simulink model "SIM_CSTR"  (R2023b)
settings: Solver=VariableStepAuto  StartTime=0.0  StopTime=30  RelTol=1e-3
values from neighbouring files (symbols this model uses):
  Ts = 0.05    [NMPC_CSTR.m]
  u0 = 300    [NMPC_CSTR.m]
libraries: sharedTrackingLibrary x1, mpclib x1, simulink x1
settings Model: Creator=DELL  LastModifiedBy=akeebismail

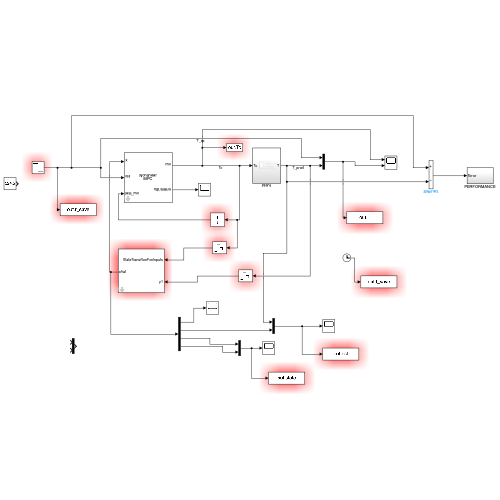
[thumbnail: Simulink's stored preview of the top-level diagram]
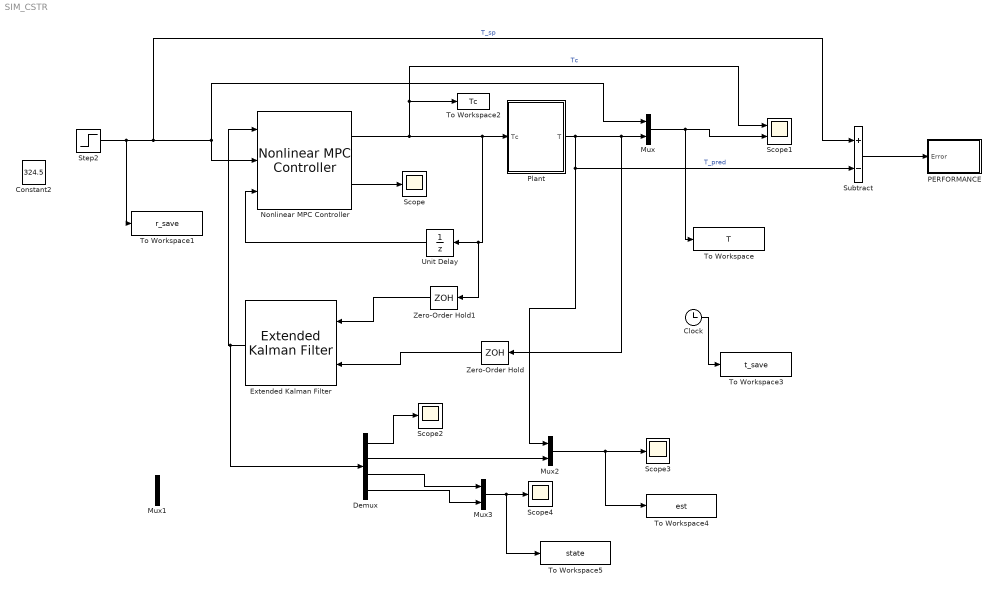
== system SIM_CSTR ==
  Clock : Clock
  Constant2 : Constant  Value=324.5
  Demux : Demux
  Extended Kalman Filter : sharedTrackingLibrary/Extended Kalman Filter  StateTransitionFcn=cstrStateFcnDT  HasStateTransitionJacobianFcn=off  HasAdditiveProcessNoise=Additive  ProcessNoise=[1e-1;1e-1;1e-1;1e-1]  HasTimeVaryingProcessNoise=off  HasStateTransitionFcnExtraArgument=1  InitialState=y0  InitialStateCovariance=[1;1;1;1]  MeasurementFcn1=cstrMeasFcn  HasMeasurementJacobianFcn1=off  HasMeasurementEnablePort1=off  HasAdditiveMeasurementNoise1=Additive  MeasurementNoise1=1e-2  HasTimeVaryingMeasurementNoise1=off  HasMeasurementFcnExtraArgument1=0  HasMeasurementWrapping1=off  MeasurementFcn2=myMeasurementFcn  HasMeasurementJacobianFcn2=off  HasMeasurementEnablePort2=off  HasAdditiveMeasurementNoise2=Additive  MeasurementNoise2=1  HasTimeVaryingMeasurementNoise2=off  HasMeasurementFcnExtraArgument2=0  HasMeasurementWrapping2=off  MeasurementFcn3=myMeasurementFcn  HasMeasurementJacobianFcn3=off  HasMeasurementEnablePort3=off  HasAdditiveMeasurementNoise3=Additive  MeasurementNoise3=1  HasTimeVaryingMeasurementNoise3=off  HasMeasurementFcnExtraArgument3=0  HasMeasurementWrapping3=off  MeasurementFcn4=myMeasurementFcn  HasMeasurementJacobianFcn4=off  HasMeasurementEnablePort4=off  HasAdditiveMeasurementNoise4=Additive  MeasurementNoise4=1  HasTimeVaryingMeasurementNoise4=off  HasMeasurementFcnExtraArgument4=0  HasMeasurementWrapping4=off  MeasurementFcn5=myMeasurementFcn  HasMeasurementJacobianFcn5=off  HasMeasurementEnablePort5=off  HasAdditiveMeasurementNoise5=Additive  MeasurementNoise5=1  HasTimeVaryingMeasurementNoise5=off  HasMeasurementFcnExtraArgument5=0  HasMeasurementWrapping5=off  EnableMultirate=off  StateTransitionFcnSampleTime=1  MeasurementFcn1SampleTime=1  MeasurementFcn2SampleTime=1  MeasurementFcn3SampleTime=1  MeasurementFcn4SampleTime=1  MeasurementFcn5SampleTime=1  UseCurrentEstimator=on  OutputStateCovariance=off  DataType=double  SampleTime=Ts  NumberOfMeasurements=1
  Mux{,1..3} (4 alike) : Mux  Inputs=2
  Nonlinear MPC Controller : mpclib/Nonlinear MPC Controller  nlmpcobj=nlobj  UseObjectTs=on  UseMEX=off  md_enabled=off  mvtarget_enabled=off  param_enabled=off  cost_enabled=off  mvseq_enabled=off  stateseq_enabled=off  ovseq_enabled=off  slack_enabled=off  status_enabled=on  ov_min=off  ov_max=off  mv_min=off  mv_max=off  mvrate_min=off  mvrate_max=off  state_min=off  state_max=off  ov_weight=off  mv_weight=off  mvrate_weight=off  ecr_weight=off  nlp_initialize=off
  PERFORMANCE : Subsystem
  Plant : Subsystem
  Scope{,2..4} (4 alike) : Scope
  Scope1 : Scope  NumInputPorts=2
  Step2 : Step  Time=10  Before=324.5  After=305  SampleTime=Ts
  Subtract : Sum  Inputs=+-
  To Workspace : ToWorkspace  VariableName=T  SaveFormat=Timeseries  SampleTime=Ts
  To Workspace1 : ToWorkspace  VariableName=r_save  SaveFormat=Timeseries  SampleTime=Ts
  To Workspace2 : ToWorkspace  VariableName=Tc  SaveFormat=Timeseries  SampleTime=Ts
  To Workspace3 : ToWorkspace  VariableName=t_save  SaveFormat=Timeseries  SampleTime=Ts
  To Workspace4 : ToWorkspace  VariableName=est  SaveFormat=Timeseries  SampleTime=Ts
  To Workspace5 : ToWorkspace  VariableName=state  SaveFormat=Timeseries  SampleTime=Ts
  Unit Delay : UnitDelay  InitialCondition=u0  SampleTime=Ts  HasFrameUpgradeWarning=on
  Zero-Order Hold : ZeroOrderHold  SampleTime=Ts
  Zero-Order Hold1 : ZeroOrderHold  SampleTime=Ts
  wires:
  Step2/1 -> To Workspace1/1, Subtract/1, Nonlinear MPC Controller/2, Mux/1  "T_sp"
  Nonlinear MPC Controller/1 -> To Workspace2/1, Scope1/1, Plant/1(Tc), Zero-Order Hold1/1, Unit Delay/1  "Tc"
  Plant/1(T) -> Subtract/2, Mux2/1, Zero-Order Hold/1, Mux/2  "T_pred"
  Nonlinear MPC Controller/2 -> Scope/1
  Mux/1 -> To Workspace/1, Scope1/2
  Zero-Order Hold/1 -> Extended Kalman Filter/2
  Unit Delay/1 -> Nonlinear MPC Controller/3
  Zero-Order Hold1/1 -> Extended Kalman Filter/1
  Clock/1 -> To Workspace3/1
  Extended Kalman Filter/1 -> Demux/1, Nonlinear MPC Controller/1
  Demux/2 -> Mux2/2
  Demux/1 -> Scope2/1
  Mux2/1 -> Scope3/1, To Workspace4/1
  Demux/3 -> Mux3/1
  Demux/4 -> Mux3/2
  Mux3/1 -> To Workspace5/1, Scope4/1
  Subtract/1 -> PERFORMANCE/1(Error)

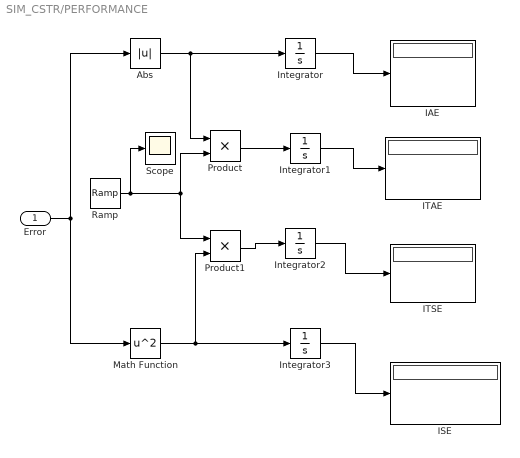
== system SIM_CSTR/PERFORMANCE ==
  Error : Inport
  Abs : Abs  SaturateOnIntegerOverflow=off
  IAE : Display
  ISE : Display
  ITAE : Display
  ITSE : Display
  Integrator{,1..3} (4 alike) : Integrator
  Math Function : Math  Operator=square  SignedPower=on
  Product : Product  RndMeth=Zero
  Product1 : Product  RndMeth=Zero
  Ramp : simulink/Sources/Ramp  slope=1  start=0  InitialOutput=0
  Scope : Scope
  wires:
  Error/1 -> Math Function/1, Abs/1
  Abs/1 -> Integrator/1, Product/1
  Integrator/1 -> IAE/1
  Ramp/1 -> Product/2, Product1/1, Scope/1
  Math Function/1 -> Integrator3/1, Product1/2
  Product1/1 -> Integrator2/1
  Product/1 -> Integrator1/1
  Integrator3/1 -> ISE/1
  Integrator2/1 -> ITSE/1
  Integrator1/1 -> ITAE/1

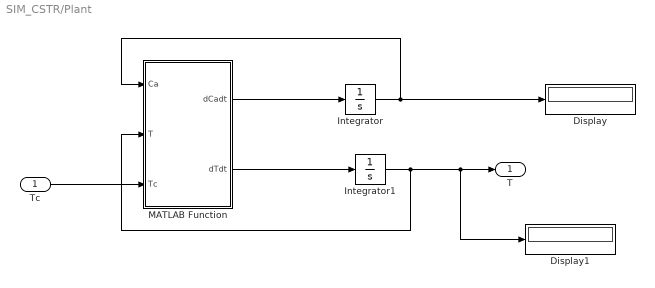
== system SIM_CSTR/Plant ==
  Tc : Inport
  Display : Display
  Display1 : Display
  Integrator : Integrator
  Integrator1 : Integrator  InitialCondition=300
  MATLAB Function : MATLAB Function  TreatAsAtomicUnit=on
  T : Outport
  wires:
  Integrator1/1 -> Display1/1, T/1, MATLAB Function/2(T)
  MATLAB Function/2(dTdt) -> Integrator1/1
  Integrator/1 -> Display/1, MATLAB Function/1(Ca)
  MATLAB Function/1(dCadt) -> Integrator/1
  Tc/1 -> MATLAB Function/3(Tc)

== matlab function SIM_CSTR/Plant/MATLAB Function ==
  data: Ca input; dCadt output; T input; Tc input; dTdt output
function [dCadt,dTdt] = fcn(Ca,T,Tc)

values = {100,5e4,350,100,1000,0.239,8750,7.2e10,5e4,1};
[F,delta_H,Tf,V,rho,Cp,E_R,k0,U_A,Caf] = values{:};

% Rate constant (Arrhenius equation)
        k = k0 * exp(-E_R / T);
        
        % Mass balance for Ca
        dCadt = F/V * (Caf - Ca) - k * Ca;
        
        % Energy balance for T
        dTdt = F/V * (Tf - T) + (delta_H / (rho * Cp)) * k * Ca + (U_A / (rho * Cp * V)) * (Tc - T);


end
